simulink model "sim_new_telemetry_system"  (R2025b)
settings: Solver=VariableStepAuto  StartTime=0.0  StopTime=10  RelTol=1e-3
model workspace (MAT data in the model file):
  tau = Simulink.Parameter
  tau.Value = 5
  tau.Complexity = 'real'
  tau.Dimensions = [1 1]
  tau.DataType = 'auto'
settings Model: Creator=strog  LastModifiedBy=strog
settings DataIOCC: SignalLogging=off

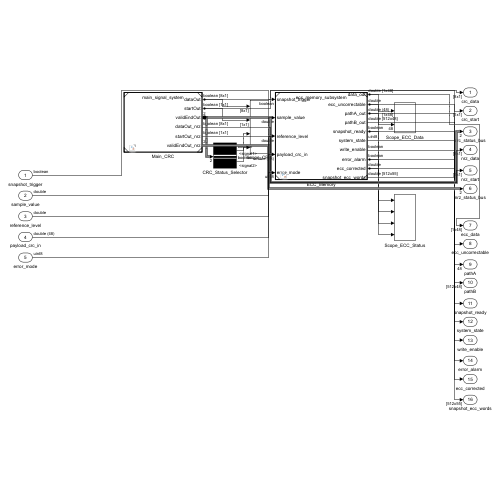
[thumbnail: Simulink's stored preview of the top-level diagram]
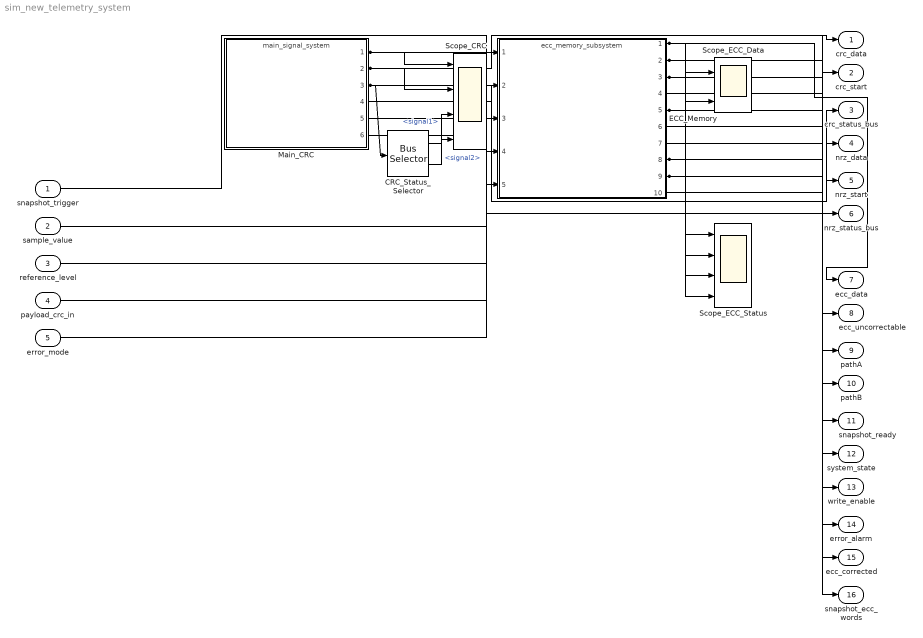
== system sim_new_telemetry_system ==
  snapshot_trigger : Inport  OutDataTypeStr=boolean  PortDimensions=1
  sample_value : Inport  Port=2  OutDataTypeStr=double  PortDimensions=1
  reference_level : Inport  Port=3  OutDataTypeStr=double  PortDimensions=1
  payload_crc_in : Inport  Port=4  OutDataTypeStr=double  PortDimensions=48
  error_mode : Inport  Port=5  OutDataTypeStr=uint8  PortDimensions=1
  CRC_Status_Selector : BusSelector  OutputSignals=signal1,signal2
  ECC_Memory : ModelReference  ModelNameDialog=ecc_memory_subsystem  SimulationMode=Normal  ModelReferenceVersion=1.17
  Main_CRC : ModelReference  ModelNameDialog=main_signal_system  SimulationMode=Normal  ModelReferenceVersion=1.25
  Scope_CRC : Scope  NumInputPorts=4
  Scope_ECC_Data : Scope  NumInputPorts=2
  Scope_ECC_Status : Scope  NumInputPorts=4
  crc_data : Outport
  crc_start : Outport  Port=2
  crc_status_bus : Outport  Port=3
  nrz_data : Outport  Port=4
  nrz_start : Outport  Port=5
  nrz_status_bus : Outport  Port=6
  ecc_data : Outport  Port=7
  ecc_uncorrectable : Outport  Port=8
  pathA : Outport  Port=9
  pathB : Outport  Port=10
  snapshot_ready : Outport  Port=11
  system_state : Outport  Port=12
  write_enable : Outport  Port=13
  error_alarm : Outport  Port=14
  ecc_corrected : Outport  Port=15
  snapshot_ecc_words : Outport  Port=16
  wires:
  Main_CRC/1 -> crc_data/1, Scope_CRC/1
  Main_CRC/2 -> crc_start/1, Scope_CRC/2
  Main_CRC/3 -> crc_status_bus/1, CRC_Status_Selector/1
  Main_CRC/4 -> nrz_data/1
  Main_CRC/5 -> nrz_start/1
  Main_CRC/6 -> nrz_status_bus/1
  ECC_Memory/1 -> ecc_data/1, Scope_ECC_Data/1
  ECC_Memory/2 -> ecc_uncorrectable/1, Scope_ECC_Status/1
  ECC_Memory/3 -> pathA/1, Scope_ECC_Data/2
  ECC_Memory/4 -> pathB/1
  ECC_Memory/5 -> snapshot_ready/1, Scope_ECC_Status/2
  ECC_Memory/6 -> system_state/1
  ECC_Memory/7 -> write_enable/1
  ECC_Memory/8 -> error_alarm/1, Scope_ECC_Status/3
  ECC_Memory/9 -> ecc_corrected/1, Scope_ECC_Status/4
  ECC_Memory/10 -> snapshot_ecc_words/1
  snapshot_trigger/1 -> ECC_Memory/1
  sample_value/1 -> ECC_Memory/2
  reference_level/1 -> ECC_Memory/3
  payload_crc_in/1 -> ECC_Memory/4
  error_mode/1 -> ECC_Memory/5
  CRC_Status_Selector/1 -> Scope_CRC/3  "<signal1>"
  CRC_Status_Selector/2 -> Scope_CRC/4  "<signal2>"
